simulink model "mVeh_fun_tbm"  (R2023b)
settings: Solver=FixedStepDiscrete  StartTime=0.0  StopTime=Parm_cnv_simulink_stopTime  FixedStep=Const_cnv_fundmt_stepSize  RelTol=1e-3  EnableMultiTasking=on
InitFcn:
  | preLoadFun
undefined symbols (not defined in the file or in its folder): Calib_pirelle_presSnr_x8, Calib_roadTriger_x6, Calib_tbm_brkBts_x8, Calib_tbm_ctr_x8, Calib_tbm_sensor_x4, Calib_tbm_strDistb_x8, Calib_tbm_supCtr_x8, CtrSet_tbm_enab_x8, IO397, Parm_tbmVeh_sig_max_numInvalid, Parm_tbmVeh_sig_tolerate_numInvalid
libraries: canmsglib x34, speedgoatlib_IO691 x19, MyLibrary x5, libtb_gen_canMsgCntr x5, speedgoatlib_fpga_analog_io x1, simulink x1, speedgoatlib_fpga x1, lib_decmp_CtrSet_tbm_enab_x8 x1, lib_decmp_Calib_tbm_brkPreTriger_x6 x1, lib_decmp_Calib_tbm_sensor_x4 x1
(part 2 of 3)

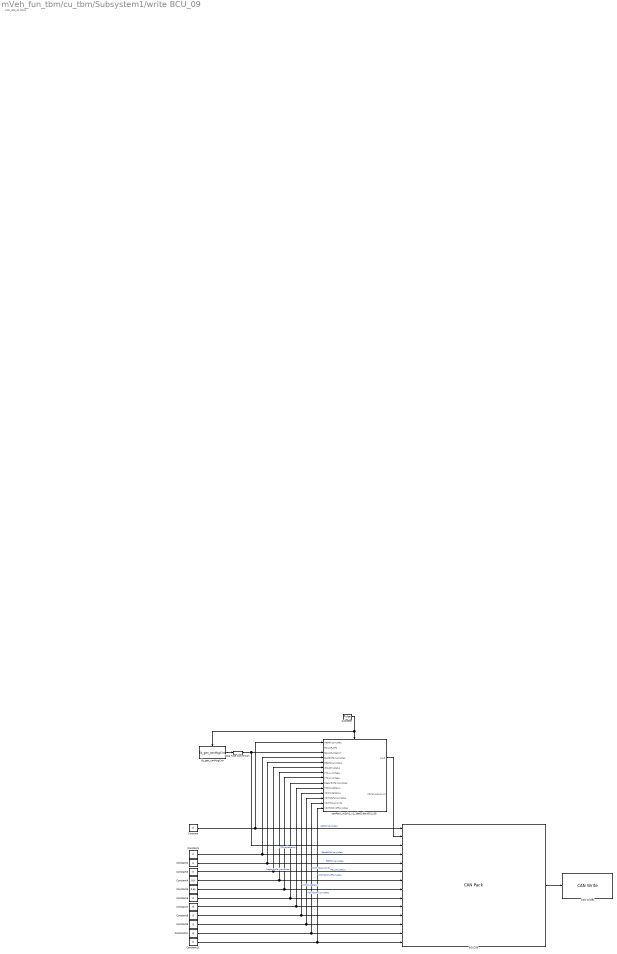
== system mVeh_fun_tbm/cu_tbm/Subsystem1/write BCU_09 ==
  note: ADC_EPS_01 20ms
  BCU_09 : canmsglib/CAN Pack  CANdbFile=C:\Users\bowen.zheng\Desktop\spdGoat_prj_20230315\spdGoat_prj_20230315\support\dbc\NIO_NT2_Chassis2_CAN_Official_Release_V_1_1_DA_02.dbc  MsgList=(none)  MsgName=BCU_09  MsgIDType=Standard (11-bit identifier)  MsgIdentifier=591  MsgLength=8  Remote=off  ApplyMinMax=off  BusOutput=off  SignalInfo={'ABSFailLampReq','37','1','BE','unsigned','Standard','0','1','0','0','1';'BCU_09_CRC','0','8','BE','unsigned','Standard','0','1','0','0','255';'BCU_09_MsgCntr','12','4','BE','unsigned','Standard','0','1','0','0','15';'BascBrkFailLampReq','32','2','BE','unsigned','Standard','0','1','0','0','3';'EBDFailLampReq','34','1','BE','unsigned','Standard','0','1','0','0','1';'IPB_CST_Status','38','2','BE','unsigned','Standard','0','1','0','0','3';'PTS_1_Voltage','17','9','BE','unsigned','Standard','0','0.01','-0.5','-0.5','4.61';'PTS_2_Voltage','24','9','BE','unsigned','Standard','0','0.01','-0.5','-0.5','4.61';'RegenBrkFailLampReq','10','1','BE','unsigned','Standard','0','1','0','0','1';'TCSModeStatus','45','3','BE','unsigned','Standard','0','1','0','0','7';'VDCModeStatus','42','3','BE','unsigned','Standard','0','1','0','0','7';'VDCTCSFailLampReq','36','1','BE','unsigned','Standard','0','1','0','0','1';'VDCTCSLampInfo','35','1','BE','unsigned','Standard','0','1','0','0','1';'VDCTCSOnOfflampReq','11','1','BE','unsigned','Standard','0','1','0','0','1'}
      settings: DataFormat=CANdb specified signals
  CAN Write1 : speedgoatlib_IO691/CAN Write  id=2  ts=0.1  channel=2  messageType=CAN  enableStatusPort=off  canType=CAN (HS)  initValues=[691 2 0.1 1 1 1 0]
  Constant{,1..3,6..11} (10 alike) : Constant  Value=0  OutDataTypeStr=single
  Constant4 : Constant  Value=0.9  OutDataTypeStr=single
  Constant5 : Constant  Value=0.44  OutDataTypeStr=single
  Data Type Conversion : DataTypeConversion  OutDataTypeStr=single  RndMeth=Nearest  SaturateOnIntegerOverflow=off
  canPack_nt2ch2_v1_1da02.dbc:BCU_09 : Subsystem
  lib_gen_canMsgCntr : libtb_gen_canMsgCntr/lib_gen_canMsgCntr  SystemSampleTime=-1  VariantActivationTime=update diagram  AllowFlexibleInterface=on  Latency=0  AutoFrameSizeCalculation=off
  pulseGen : DiscretePulseGenerator  PulseType=Time based  Period=0.1  PulseWidth=50
  wires:
  BCU_09/1 -> CAN Write1/1
  lib_gen_canMsgCntr/1 -> Data Type Conversion/1
  Constant/1 -> canPack_nt2ch2_v1_1da02.dbc:BCU_09/1(ABSFailLampReq), BCU_09/1  "ABSFailLampReq"
  Constant1/1 -> canPack_nt2ch2_v1_1da02.dbc:BCU_09/4(BascBrkFailLampReq), BCU_09/4  "BascBrkFailLampReq"
  Constant2/1 -> canPack_nt2ch2_v1_1da02.dbc:BCU_09/5(EBDFailLampReq), BCU_09/5  "EBDFailLampReq"
  Constant3/1 -> canPack_nt2ch2_v1_1da02.dbc:BCU_09/6(IPB_CST_Status), BCU_09/6  "IPB_CST_Status"
  Constant4/1 -> canPack_nt2ch2_v1_1da02.dbc:BCU_09/7(PTS_1_Voltage), BCU_09/7
  Constant5/1 -> canPack_nt2ch2_v1_1da02.dbc:BCU_09/8(PTS_2_Voltage), BCU_09/8
  Constant6/1 -> canPack_nt2ch2_v1_1da02.dbc:BCU_09/9(RegenBrkFailLampReq), BCU_09/9  "RegenBrkFailLampReq"
  Constant7/1 -> canPack_nt2ch2_v1_1da02.dbc:BCU_09/10(TCSModeStatus), BCU_09/10  "TCSModeStatus"
  Constant8/1 -> canPack_nt2ch2_v1_1da02.dbc:BCU_09/11(VDCModeStatus), BCU_09/11  "VDCModeStatus"
  Constant9/1 -> BCU_09/12, canPack_nt2ch2_v1_1da02.dbc:BCU_09/12(VDCTCSFailLampReq)  "VDCTCSFailLampReq"
  Constant10/1 -> canPack_nt2ch2_v1_1da02.dbc:BCU_09/13(VDCTCSLampInfo), BCU_09/13  "VDCTCSLampInfo"
  Constant11/1 -> canPack_nt2ch2_v1_1da02.dbc:BCU_09/14(VDCTCSOnOfflampReq), BCU_09/14  "VDCTCSOnOfflampReq"
  pulseGen/1 -> lib_gen_canMsgCntr/Trigger, canPack_nt2ch2_v1_1da02.dbc:BCU_09/Trigger
  Data Type Conversion/1 -> BCU_09/3, canPack_nt2ch2_v1_1da02.dbc:BCU_09/3(BCU_09_MsgCntr)
  canPack_nt2ch2_v1_1da02.dbc:BCU_09/1(crc_8) -> BCU_09/2

== system mVeh_fun_tbm/cu_tbm/Subsystem1/write VCU_14 ==
  note: ADC_EPS_01 20ms
  note: VCU_14 10ms
  cmd_brk_4whPres : Inport
  Bus Selector : BusSelector  OutputSignals=BTS_Active,BTS_BrakeTar_FL,BTS_BrakeTar_FR,BTS_BrakeTar_RL,BTS_BrakeTar_RR,VCU_14_CRC,VCU_14_MsgCntr
  CAN Write1 : speedgoatlib_IO691/CAN Write  id=2  ts=0.01  channel=2  messageType=CAN  enableStatusPort=off  canType=CAN (HS)  initValues=[691 2 0.01 1 1 1 0]
  Data Type Conversion : DataTypeConversion  OutDataTypeStr=single  RndMeth=Nearest  SaturateOnIntegerOverflow=off
  VCU_14*1 : canmsglib/CAN Pack  CANdbFile=.\support\dbc\NIO_NT2_Chassis2_CAN_Official_Release_V_1_1_DA_02.dbc  MsgList=VCU_14  MsgName=VCU_14  MsgIDType=Standard (11-bit identifier)  MsgIdentifier=75  MsgLength=8  Remote=off  ApplyMinMax=off  BusOutput=off  SignalInfo={'BTS_Active','23','1','BE','unsigned','Standard','0','1','0','0','1';'BTS_BrakeTar_FL','16','7','BE','unsigned','Standard','0','1','0','0','127';'BTS_BrakeTar_FR','25','7','BE','unsigned','Standard','0','1','0','0','127';'BTS_BrakeTar_RL','34','7','BE','unsigned','Standard','0','1','0','0','127';'BTS_BrakeTar_RR','43','7','BE','unsigned','Standard','0','1','0','0','127';'VCU_14_CRC','0','8','BE','unsigned','Standard','0','1','0','0','255';'VCU_14_MsgCntr','12','4','BE','unsigned','Standard','0','1','0','0','15'}
      settings: DataFormat=CANdb specified signals
  canPack_nt2ch2_v1_1da02.dbc:VCU_14 : Subsystem
  lib_gen_canMsgCntr : libtb_gen_canMsgCntr/lib_gen_canMsgCntr  SystemSampleTime=-1  VariantActivationTime=update diagram  AllowFlexibleInterface=on  Latency=0  AutoFrameSizeCalculation=off
  pulseGen : DiscretePulseGenerator  PulseType=Time based  Period=0.01  PulseWidth=50
  wires:
  canPack_nt2ch2_v1_1da02.dbc:VCU_14/1(crc_8) -> VCU_14*1/6
  VCU_14*1/1 -> CAN Write1/1
  cmd_brk_4whPres/1 -> Bus Selector/1
  pulseGen/1 -> canPack_nt2ch2_v1_1da02.dbc:VCU_14/Trigger, lib_gen_canMsgCntr/Trigger
  lib_gen_canMsgCntr/1 -> Data Type Conversion/1
  Bus Selector/1 -> canPack_nt2ch2_v1_1da02.dbc:VCU_14/1(BTS_Active), VCU_14*1/1  "<BTS_Active>"
  Bus Selector/6 -> ?  "<VCU_14_CRC>"
  Bus Selector/7 -> ?  "<VCU_14_MsgCntr>"
  Data Type Conversion/1 -> canPack_nt2ch2_v1_1da02.dbc:VCU_14/7(VCU_14_MsgCntr), VCU_14*1/7
  Bus Selector/2 -> canPack_nt2ch2_v1_1da02.dbc:VCU_14/2(BTS_BrakeTar_FL), VCU_14*1/2  "<BTS_BrakeTar_FL>"
  Bus Selector/3 -> canPack_nt2ch2_v1_1da02.dbc:VCU_14/3(BTS_BrakeTar_FR), VCU_14*1/3  "<BTS_BrakeTar_FR>"
  Bus Selector/4 -> canPack_nt2ch2_v1_1da02.dbc:VCU_14/4(BTS_BrakeTar_RL), VCU_14*1/4  "<BTS_BrakeTar_RL>"
  Bus Selector/5 -> canPack_nt2ch2_v1_1da02.dbc:VCU_14/5(BTS_BrakeTar_RR), VCU_14*1/5  "<BTS_BrakeTar_RR>"

== system mVeh_fun_tbm/cu_tbm/asm_canMsg/to_bcu_bts ==
  bts_enab : Inport
  cu_tbm : Inport  Port=2
  Bus Selector : BusSelector  OutputSignals=btsSimuDrBrk_actv,btsSimuDrBrk_mcp,tbmModfBrk_actv_4w,tbmModfBrk_pTgt_4w
  Data Type Conversion : DataTypeConversion  OutDataTypeStr=single  RndMeth=Nearest  SaturateOnIntegerOverflow=off
  Demux : Demux
  MATLAB Function : MATLAB Function  TreatAsAtomicUnit=on
  Rate Transition : RateTransition
  bus_VCU_14 : BusCreator  Inputs=7
  bus_to_ch2_VCU_14 : Outport
  wires:
  cu_tbm/1 -> Bus Selector/1
  ? -> bus_VCU_14/6  "VCU_14_CRC"
  ? -> bus_VCU_14/7  "VCU_14_MsgCntr"
  Demux/1 -> bus_VCU_14/2  "BTS_BrakeTar_FL"
  Demux/3 -> bus_VCU_14/4  "BTS_BrakeTar_RL"
  Data Type Conversion/1 -> bus_VCU_14/1  "BTS_Active"
  bus_VCU_14/1 -> bus_to_ch2_VCU_14/1  "bus_to_ch2_VCU_14"
  Demux/2 -> bus_VCU_14/3  "BTS_BrakeTar_FR"
  Demux/4 -> bus_VCU_14/5  "BTS_BrakeTar_RR"
  Bus Selector/1 -> MATLAB Function/2(btsSimuDrBrk_actv)  "<btsSimuDrBrk_actv>"
  MATLAB Function/1(btsCtr_actv) -> Rate Transition/1
  Bus Selector/3 -> MATLAB Function/4(tbmModfBrk_actv_4w)  "<tbmModfBrk_actv_4w>"
  Bus Selector/4 -> MATLAB Function/5(tbmModfBrk_pTgt_4w)  "<tbmModfBrk_pTgt_4w>"
  Bus Selector/2 -> MATLAB Function/3(btsSimuDrBrk_pTgt_4w)  "<btsSimuDrBrk_mcp>"
  MATLAB Function/2(bts_pTgt_4w) -> Demux/1  "bts_pTgt_4w"
  bts_enab/1 -> MATLAB Function/1(bts_enab)
  Rate Transition/1 -> Data Type Conversion/1

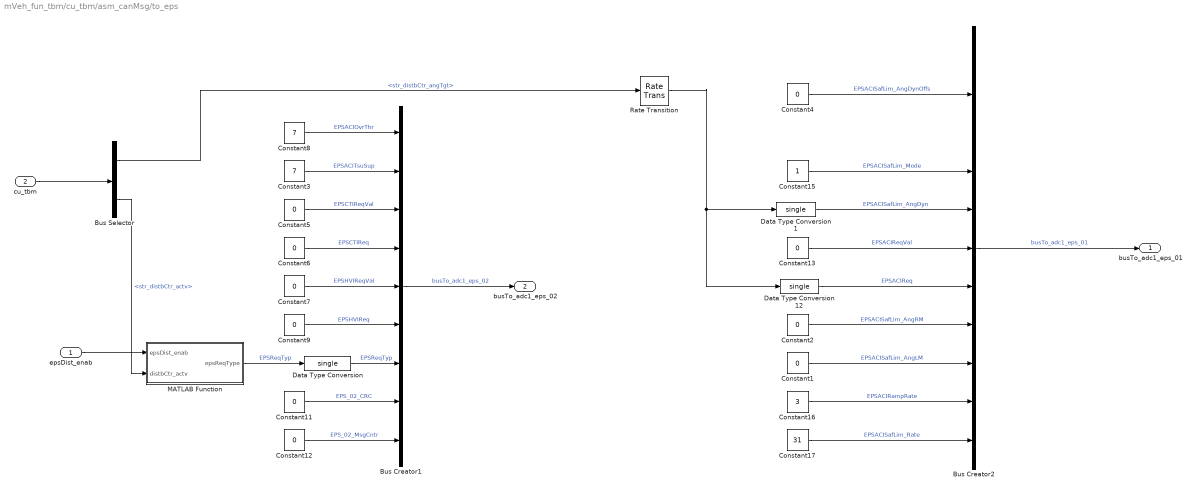
== system mVeh_fun_tbm/cu_tbm/asm_canMsg/to_eps ==
  epsDist_enab : Inport
  cu_tbm : Inport  Port=2
  Bus Creator1 : BusCreator  Inputs=9
  Bus Creator2 : BusCreator  Inputs=11
  Bus Selector : BusSelector  OutputSignals=str_distbCtr_angTgt,str_distbCtr_actv
  Constant{1..2,4..7,9,11..13} (10 alike) : Constant  Value=0  OutDataTypeStr=single
  Constant15 : Constant  OutDataTypeStr=single
  Constant16 : Constant  Value=3  OutDataTypeStr=single
  Constant17 : Constant  Value=31  OutDataTypeStr=single
  Constant3 : Constant  Value=7  OutDataTypeStr=single
  Constant8 : Constant  Value=7  OutDataTypeStr=single
  Data Type Conversion : DataTypeConversion  OutDataTypeStr=single  RndMeth=Nearest  SaturateOnIntegerOverflow=off
  Data Type Conversion1 : DataTypeConversion  OutDataTypeStr=single  RndMeth=Nearest  SaturateOnIntegerOverflow=off
  Data Type Conversion12 : DataTypeConversion  OutDataTypeStr=single  RndMeth=Nearest  SaturateOnIntegerOverflow=off
  MATLAB Function : MATLAB Function  TreatAsAtomicUnit=on
  Rate Transition : RateTransition
  busTo_adc1_eps_01 : Outport
  busTo_adc1_eps_02 : Outport  Port=2
  wires:
  ? -> Bus Creator2/3  "EPS_01_MsgCntr"
  Bus Selector/1 -> Rate Transition/1  "<str_distbCtr_angTgt>"
  Constant9/1 -> Bus Creator1/6  "EPSHVIReq"
  Constant11/1 -> Bus Creator1/8  "EPS_02_CRC"
  ? -> Bus Creator2/1  "EPS_01_CRC"
  Constant2/1 -> Bus Creator2/8  "EPSACISafLim_AngRM"
  MATLAB Function/1(epsReqType) -> Data Type Conversion/1  "EPSReqTyp"
  Constant17/1 -> Bus Creator2/11  "EPSACISafLim_Rate"
  Data Type Conversion1/1 -> Bus Creator2/5  "EPSACISafLim_AngDyn"
  Constant12/1 -> Bus Creator1/9  "EPS_02_MsgCntr"
  Constant1/1 -> Bus Creator2/9  "EPSACISafLim_AngLM"
  Bus Creator2/1 -> busTo_adc1_eps_01/1  "busTo_adc1_eps_01"
  Constant7/1 -> Bus Creator1/5  "EPSHVIReqVal"
  Constant6/1 -> Bus Creator1/4  "EPSCTIReq"
  Data Type Conversion12/1 -> Bus Creator2/7  "EPSACIReq"
  Constant13/1 -> Bus Creator2/6  "EPSACIReqVal"
  Constant16/1 -> Bus Creator2/10  "EPSACIRampRate"
  Constant3/1 -> Bus Creator1/2  "EPSACITsuSup"
  Constant8/1 -> Bus Creator1/1  "EPSACIOvrThr"
  Bus Creator1/1 -> busTo_adc1_eps_02/1  "busTo_adc1_eps_02"
  Constant5/1 -> Bus Creator1/3  "EPSCTIReqVal"
  Constant4/1 -> Bus Creator2/2  "EPSACISafLim_AngDynOffs"
  Constant15/1 -> Bus Creator2/4  "EPSACISafLim_Mode"
  cu_tbm/1 -> Bus Selector/1
  Bus Selector/2 -> MATLAB Function/2(distbCtr_actv)  "<str_distbCtr_actv>"
  epsDist_enab/1 -> MATLAB Function/1(epsDist_enab)
  Data Type Conversion/1 -> Bus Creator1/7  "EPSReqTyp"
  Rate Transition/1 -> Data Type Conversion12/1, Data Type Conversion1/1

== system mVeh_fun_tbm/cu_tbm/asm_canMsg/to_suspension ==
  suspCtr_enab : Inport
  cu_tbm : Inport  Port=2
  0: dump 2whls simutaniously : Constant  Value=0  OutDataTypeStr=single
  Bus Creator : BusCreator  Inputs=10
  Bus Selector : BusSelector  OutputSignals=susp_ctrActv_4w,susp_pTgt_4w
  Constant1 : Constant  Value=0  OutDataTypeStr=single
  Demux : Demux
  Demux1 : Demux
  MATLAB Function : MATLAB Function  TreatAsAtomicUnit=on
  RT{1..2,4..5} (4 alike) : RateTransition  OutPortSampleTime=0.001
  busTo_ch1_tbm_02 : Outport
  wires:
  cu_tbm/1 -> Bus Selector/1
  0: dump 2whls simutaniously/1 -> Bus Creator/5  "springID"
  Demux1/4 -> Bus Creator/4  "LeakActv_spring4"
  Demux/2 -> Bus Creator/7  "LeakTargPres_spring2"
  Demux/3 -> Bus Creator/8  "LeakTargPres_spring3"
  Demux/4 -> Bus Creator/9  "LeakTargPres_spring4"
  Demux1/1 -> Bus Creator/1  "LeakActv_spring1"
  Constant1/1 -> Bus Creator/10  "reserved"
  Demux1/2 -> Bus Creator/2  "LeakActv_spring2"
  Demux1/3 -> Bus Creator/3  "LeakActv_spring3"
  Demux/1 -> Bus Creator/6  "LeakTargPres_spring1"
  Bus Creator/1 -> busTo_ch1_tbm_02/1  "busTo_ch1_tbm_02"
  Bus Selector/2 -> RT5/1  "<susp_pTgt_4w>"
  Bus Selector/1 -> RT1/1  "<susp_ctrActv_4w>"
  MATLAB Function/1(suspCtr_actv_4w) -> RT4/1
  suspCtr_enab/1 -> RT2/1
  RT2/1 -> MATLAB Function/1(suspCtr_enab)
  RT1/1 -> MATLAB Function/2(suspCtr_actv_4w_in)
  RT5/1 -> Demux/1
  RT4/1 -> Demux1/1

== system mVeh_fun_tbm/cu_tbm/CAN Receive Unpack/Subsystem/ADC_Waypoint1 ==
  In1 : Inport
  ADC_Waypoint01 : canmsglib/CAN Unpack  CANdbFile=C:\Users\bowen.zheng\Desktop\spdGoat_prj_20230605\spdGoat_prj_20230605\support\dbc\NIO_NT2_Chassis2_CAN_Official_Release_V_1_1_DA_02.dbc  MsgList=ADC1_WayPoint01  MsgName=ADC1_WayPoint01  MsgIDType=Standard (11-bit identifier)  MsgIdentifier=214  MsgLength=8  SignalInfo={'LD_Confidence_1','24','4','BE','unsigned','Standard','0','0.1','0','0','1.5';'LD_First_End_1','51','7','BE','unsigned','Standard','0','1','0','0','127';'LD_First_Start_1','16','8','BE','unsigned','Standard','0','0.1','0','0','25.5';'LD_First_Type_1','28','4','BE','unsigned','Standard','0','1','0','0','15';'LD_Line_First_C0_1','56','11','BE','unsigned','Standard','0','0.01','-10.24','-10.24','10.23';'LD_Line_First_C1_1','43','13','BE','unsigned','Standard','0','0.0001','-0.4096','-0.4096','0.4095';'LD_Line_First_C2_1','0','8','BE','unsigned','Standard','0','0.0001','-0.0128','-0.0128','0.0127';'LD_Line_First_C3_1','8','8','BE','unsigned','Standard','0','1e-06','-0.000128','-0.000128','0.000127'}  IDPort=off  TimestampPort=off  ErrorPort=off  RemotePort=off  LengthPort=off  StatusPort=off  ApplyMinMax=off
      settings: DataFormat=CANdb specified signals
  LD_Confidence_1 : Outport
  LD_Line_First_C0_1 : Outport  Port=2
  wires:
  In1/1 -> ADC_Waypoint01/1
  ADC_Waypoint01/1 -> LD_Confidence_1/1  "LD_Confidence_1"
  ADC_Waypoint01/5 -> LD_Line_First_C0_1/1  "LD_Line_First_C0_1"

== system mVeh_fun_tbm/cu_tbm/CAN Receive Unpack/Subsystem/ADC_Waypoint2 ==
  In1 : Inport
  ADC_Waypoint01 : canmsglib/CAN Unpack  CANdbFile=C:\Users\bowen.zheng\Desktop\spdGoat_prj_20230605\spdGoat_prj_20230605\support\dbc\NIO_NT2_Chassis2_CAN_Official_Release_V_1_1_DA_02.dbc  MsgList=ADC1_WayPoint02  MsgName=ADC1_WayPoint02  MsgIDType=Standard (11-bit identifier)  MsgIdentifier=215  MsgLength=8  SignalInfo={'LD_Confidence_2','24','4','BE','unsigned','Standard','0','0.1','0','0','1.5';'LD_First_End_2','51','7','BE','unsigned','Standard','0','1','0','0','127';'LD_First_Start_2','16','8','BE','unsigned','Standard','0','0.1','0','0','25.5';'LD_First_Type_2','28','4','BE','unsigned','Standard','0','1','0','0','15';'LD_Line_First_C0_2','56','11','BE','unsigned','Standard','0','0.01','-10.24','-10.24','10.23';'LD_Line_First_C1_2','43','13','BE','unsigned','Standard','0','0.0001','-0.4096','-0.4096','0.4095';'LD_Line_First_C2_2','0','8','BE','unsigned','Standard','0','0.0001','-0.0128','-0.0128','0.0127';'LD_Line_First_C3_2','8','8','BE','unsigned','Standard','0','1e-06','-0.000128','-0.000128','0.000127'}  IDPort=off  TimestampPort=off  ErrorPort=off  RemotePort=off  LengthPort=off  StatusPort=off  ApplyMinMax=off
      settings: DataFormat=CANdb specified signals
  LD_Confidence_2 : Outport
  LD_Line_First_C0_2 : Outport  Port=2
  wires:
  In1/1 -> ADC_Waypoint01/1
  ADC_Waypoint01/1 -> LD_Confidence_2/1  "LD_Confidence_2"
  ADC_Waypoint01/5 -> LD_Line_First_C0_2/1  "LD_Line_First_C0_2"

== system mVeh_fun_tbm/cu_tbm/CAN Receive Unpack/Subsystem/ADC_Waypoint3 ==
  In1 : Inport
  ADC_Waypoint01 : canmsglib/CAN Unpack  CANdbFile=C:\Users\bowen.zheng\Desktop\spdGoat_prj_20230605\spdGoat_prj_20230605\support\dbc\NIO_NT2_Chassis2_CAN_Official_Release_V_1_1_DA_02.dbc  MsgList=ADC1_WayPoint03  MsgName=ADC1_WayPoint03  MsgIDType=Standard (11-bit identifier)  MsgIdentifier=216  MsgLength=8  SignalInfo={'LD_Confidence_3','24','4','BE','unsigned','Standard','0','0.1','0','0','1.5';'LD_First_End_3','51','7','BE','unsigned','Standard','0','1','0','0','127';'LD_First_Start_3','16','8','BE','unsigned','Standard','0','0.1','0','0','25.5';'LD_First_Type_3','28','4','BE','unsigned','Standard','0','1','0','0','15';'LD_Line_First_C0_3','56','11','BE','unsigned','Standard','0','0.01','-10.24','-10.24','10.23';'LD_Line_First_C1_3','43','13','BE','unsigned','Standard','0','0.0001','-0.4096','-0.4096','0.4095';'LD_Line_First_C2_3','0','8','BE','unsigned','Standard','0','0.0001','-0.0128','-0.0128','0.0127';'LD_Line_First_C3_3','8','8','BE','unsigned','Standard','0','1e-06','-0.000128','-0.000128','0.000127'}  IDPort=off  TimestampPort=off  ErrorPort=off  RemotePort=off  LengthPort=off  StatusPort=off  ApplyMinMax=off
      settings: DataFormat=CANdb specified signals
  LD_Confidence_3 : Outport
  LD_Line_First_C0_3 : Outport  Port=2
  wires:
  In1/1 -> ADC_Waypoint01/1
  ADC_Waypoint01/1 -> LD_Confidence_3/1  "LD_Confidence_3"
  ADC_Waypoint01/5 -> LD_Line_First_C0_3/1  "LD_Line_First_C0_3"

== system mVeh_fun_tbm/cu_tbm/CAN Receive Unpack/Subsystem/ADC_Waypoint4 ==
  In1 : Inport
  ADC_Waypoint01 : canmsglib/CAN Unpack  CANdbFile=C:\Users\bowen.zheng\Desktop\spdGoat_prj_20230605\spdGoat_prj_20230605\support\dbc\NIO_NT2_Chassis2_CAN_Official_Release_V_1_1_DA_02.dbc  MsgList=ADC1_WayPoint04  MsgName=ADC1_WayPoint04  MsgIDType=Standard (11-bit identifier)  MsgIdentifier=217  MsgLength=8  SignalInfo={'LD_Confidence_4','24','4','BE','unsigned','Standard','0','0.1','0','0','1.5';'LD_First_End_4','51','7','BE','unsigned','Standard','0','1','0','0','127';'LD_First_Start_4','16','8','BE','unsigned','Standard','0','0.1','0','0','25.5';'LD_First_Type_4','28','4','BE','unsigned','Standard','0','1','0','0','15';'LD_Line_First_C0_4','56','11','BE','unsigned','Standard','0','0.01','-10.24','-10.24','10.23';'LD_Line_First_C1_4','43','13','BE','unsigned','Standard','0','0.0001','-0.4096','-0.4096','0.4095';'LD_Line_First_C2_4','0','8','BE','unsigned','Standard','0','0.0001','-0.0128','-0.0128','0.0127';'LD_Line_First_C3_4','8','8','BE','unsigned','Standard','0','1e-06','-0.000128','-0.000128','0.000127'}  IDPort=off  TimestampPort=off  ErrorPort=off  RemotePort=off  LengthPort=off  StatusPort=off  ApplyMinMax=off
      settings: DataFormat=CANdb specified signals
  LD_Confidence_4 : Outport
  LD_Line_First_C0_4 : Outport  Port=2
  wires:
  In1/1 -> ADC_Waypoint01/1
  ADC_Waypoint01/1 -> LD_Confidence_4/1  "LD_Confidence_4"
  ADC_Waypoint01/5 -> LD_Line_First_C0_4/1  "LD_Line_First_C0_4"

== system mVeh_fun_tbm/cu_tbm/Chassis 1 read/Subsystem/ACM_02 ==
  In1 : Inport
  Chassis 1 ACM_02 : canmsglib/CAN Unpack  CANdbFile=.\support\dbc\NIO_NT2_Chassis1_CAN_Official_Release_V_1_1_DA_02.dbc  MsgList=ACM_02  MsgName=ACM_02  MsgIDType=Standard (11-bit identifier)  MsgIdentifier=61  MsgLength=6  SignalInfo={'ACM_02_CRC','0','8','BE','unsigned','Standard','0','1','0','0','255';'ACM_02_MsgCntr','12','4','BE','unsigned','Standard','0','1','0','0','15';'LatA','40','16','BE','unsigned','Standard','0','0.001','-2','-2','2';'LatAValSts','8','2','BE','unsigned','Standard','0','1','0','0','3';'YawRate','24','16','BE','unsigned','Standard','0','0.01','-180','-180','180';'YawRateValSts','10','2','BE','unsigned','Standard','0','1','0','0','3'}  IDPort=off  TimestampPort=off  ErrorPort=off  RemotePort=off  LengthPort=off  StatusPort=off  ApplyMinMax=off
      settings: DataFormat=CANdb specified signals
  Terminator : Terminator
  Terminator1 : Terminator
  wires:
  In1/1 -> Chassis 1 ACM_02/1
  Chassis 1 ACM_02/3 -> Terminator/1  "ACM_02_LatA"
  Chassis 1 ACM_02/5 -> Terminator1/1  "ACM_02_YawRate"

== system mVeh_fun_tbm/cu_tbm/Chassis 1 read/Subsystem/ACM_03 ==
  In1 : Inport
  Chassis 1 ACM_03 : canmsglib/CAN Unpack  CANdbFile=.\support\dbc\NIO_NT2_Chassis1_CAN_Official_Release_V_1_1_DA_02.dbc  MsgList=ACM_03  MsgName=ACM_03  MsgIDType=Standard (11-bit identifier)  MsgIdentifier=62  MsgLength=4  SignalInfo={'ACM_03_CRC','0','8','BE','unsigned','Standard','0','1','0','0','255';'ACM_03_MsgCntr','12','4','BE','unsigned','Standard','0','1','0','0','15';'AxAyYrsCalSts','8','2','BE','unsigned','Standard','0','1','0','0','3';'LgtA','24','16','BE','unsigned','Standard','0','0.001','-2','-2','2';'LgtAValSts','10','2','BE','unsigned','Standard','0','1','0','0','3'}  IDPort=off  TimestampPort=off  ErrorPort=off  RemotePort=off  LengthPort=off  StatusPort=off  ApplyMinMax=off
      settings: DataFormat=CANdb specified signals
  Terminator1 : Terminator
  wires:
  In1/1 -> Chassis 1 ACM_03/1
  Chassis 1 ACM_03/4 -> Terminator1/1  "ACM_03_LgtA"

== system mVeh_fun_tbm/cu_tbm/Chassis 1 read/Subsystem/BCU_01 ==
  In1 : Inport
  Chassis 1 BCU_01 : canmsglib/CAN Unpack  CANdbFile=.\support\dbc\NIO_NT2_Chassis1_CAN_Official_Release_V_1_1_DA_02.dbc  MsgList=BCU_01  MsgName=BCU_01  MsgIDType=Standard (11-bit identifier)  MsgIdentifier=88  MsgLength=6  SignalInfo={'BCU_01_CRC','0','8','BE','unsigned','Standard','0','1','0','0','255';'BCU_01_MsgCntr','12','4','BE','unsigned','Standard','0','1','0','0','15';'WhlSpdFrntLe','24','13','BE','unsigned','Standard','0','0.05625','0','0','360';'WhlSpdFrntLeMovgDir','37','2','BE','unsigned','Standard','0','1','0','0','3';'WhlSpdFrntLeSts','10','2','BE','unsigned','Standard','0','1','0','0','3';'WhlSpdFrntRi','40','13','BE','unsigned','Standard','0','0.05625','0','0','360';'WhlSpdFrntRiMovgDir','21','2','BE','unsigned','Standard','0','1','0','0','3';'WhlSpdFrntRiSts','8','2','BE','unsigned','Standard','0','1','0','0','3'}  IDPort=off  TimestampPort=off  ErrorPort=off  RemotePort=off  LengthPort=off  StatusPort=off  ApplyMinMax=off
      settings: DataFormat=CANdb specified signals
  Terminator1 : Terminator
  Terminator2 : Terminator
  wires:
  In1/1 -> Chassis 1 BCU_01/1
  Chassis 1 BCU_01/3 -> Terminator2/1  "BCU_01_WhlSpdFrntLe"
  Chassis 1 BCU_01/6 -> Terminator1/1  "BCU_01_WhlSpdFrntRi"

== system mVeh_fun_tbm/cu_tbm/Chassis 1 read/Subsystem/BCU_02 ==
  In1 : Inport
  Chassis 1 BCU_02 : canmsglib/CAN Unpack  CANdbFile=.\support\dbc\NIO_NT2_Chassis1_CAN_Official_Release_V_1_1_DA_02.dbc  MsgList=BCU_02  MsgName=BCU_02  MsgIDType=Standard (11-bit identifier)  MsgIdentifier=89  MsgLength=6  SignalInfo={'BCU_02_CRC','0','8','BE','unsigned','Standard','0','1','0','0','255';'BCU_02_MsgCntr','12','4','BE','unsigned','Standard','0','1','0','0','15';'WhlSpdReLe','24','13','BE','unsigned','Standard','0','0.05625','0','0','360';'WhlSpdReLeMovgDir','21','2','BE','unsigned','Standard','0','1','0','0','3';'WhlSpdReLeSts','10','2','BE','unsigned','Standard','0','1','0','0','3';'WhlSpdReRi','40','13','BE','unsigned','Standard','0','0.05625','0','0','360';'WhlSpdReRiMovgDir','37','2','BE','unsigned','Standard','0','1','0','0','3';'WhlSpdReRiSts','8','2','BE','unsigned','Standard','0','1','0','0','3'}  IDPort=off  TimestampPort=off  ErrorPort=off  RemotePort=off  LengthPort=off  StatusPort=off  ApplyMinMax=off
      settings: DataFormat=CANdb specified signals
  Terminator1 : Terminator
  Terminator2 : Terminator
  wires:
  In1/1 -> Chassis 1 BCU_02/1
  Chassis 1 BCU_02/3 -> Terminator2/1  "BCU_02_WhlSpdReLe"
  Chassis 1 BCU_02/6 -> Terminator1/1  "BCU_02_WhlSpdReRi"

== system mVeh_fun_tbm/cu_tbm/Chassis 1 read/Subsystem/BCU_04 ==
  In1 : Inport
  Bus Creator : BusCreator  Inputs=2
  Bus Creator1 : BusCreator  Inputs=2
  Chassis 1 BCU_04 : canmsglib/CAN Unpack  CANdbFile=.\support\dbc\NIO_NT2_Chassis1_CAN_Official_Release_V_1_1_DA_02.dbc  MsgList=BCU_04  MsgName=BCU_04  MsgIDType=Standard (11-bit identifier)  MsgIdentifier=91  MsgLength=8  SignalInfo={'BCUBrkLiReq','9','2','BE','unsigned','Standard','0','1','0','0','3';'BCU_04_CRC','0','8','BE','unsigned','Standard','0','1','0','0','255';'BCU_04_MsgCntr','12','4','BE','unsigned','Standard','0','1','0','0','15';'BCU_NoBrkF','8','1','BE','unsigned','Standard','0','1','0','0','1';'BCU_SupInfo','48','2','BE','unsigned','Standard','0','1','0','0','3';'BrkOverHeat','50','1','BE','unsigned','Standard','0','1','0','0','1';'BrkPedlSts','54','2','BE','unsigned','Standard','0','1','0','0','3';'BrkPedlTrvl','56','8','BE','unsigned','Standard','0','0.4','0','0','102';'BrkPedlTrvlCalSts','52','2','BE','unsigned','Standard','0','1','0','0','3';'BrkPress','47','9','BE','unsigned','Standard','0','1','-42.5','-42.5','425.5';'BrkPressOffset','42','5','BE','unsigned','Standard','0','1','-15','-15','15';'BrkPressOffsetValid','41','1','BE','unsigned','Standard','0','1','0','0','1';'BrkPressValid','40','1','BE','unsigned','Standard','0','1','0','0','1';'HAZReq','11','1','BE','unsigned','Standard','0','1','0','0','1';'IPB_TwoFoot_DriveWarning','51','1','BE','unsigned','Standard','0','1','0','0','1';'VehMovgDir','21','2','BE','unsigned','Standard','0','1','0','0','3';'VehSpd','24','13','BE','unsigned','Standard','0','0.05625','0','0','360';'VehSpdSts','23','1','BE','unsigned','Standard','0','1','0','0','1'}  IDPort=off  TimestampPort=off  ErrorPort=off  RemotePort=off  LengthPort=off  StatusPort=off  ApplyMinMax=off
      settings: DataFormat=CANdb specified signals
  Terminator{,1..4} (5 alike) : Terminator
  BCU_04_VehSpd_w_Validity : Outport
  BCU_04_BrkPedl_w_Sts : Outport  Port=2
  wires:
  Chassis 1 BCU_04/8 -> Terminator2/1  "BCU_04_BrkPedlTrvl"
  Chassis 1 BCU_04/3 -> Terminator/1  "BCU_04_MsgCntr"
  Chassis 1 BCU_04/2 -> Terminator1/1  "BCU_04_CRC"
  Chassis 1 BCU_04/7 -> Bus Creator1/1  "BCU_04_BrkPedlSts"
  Chassis 1 BCU_04/13 -> Terminator4/1  "BCU_04_BrkPressValid"
  Chassis 1 BCU_04/10 -> Terminator3/1  "BCU_04_BrkPress"
  Chassis 1 BCU_04/17 -> Bus Creator/1  "BCU_04_VehSpd"
  Chassis 1 BCU_04/18 -> Bus Creator/2  "BCU_04_VehSpdSts"
  Chassis 1 BCU_04/9 -> Bus Creator1/2  "BCU_04_BrkPedlTrvlCalSts"
  In1/1 -> Chassis 1 BCU_04/1
  Bus Creator/1 -> BCU_04_VehSpd_w_Validity/1
  Bus Creator1/1 -> BCU_04_BrkPedl_w_Sts/1

== system mVeh_fun_tbm/cu_tbm/Chassis 1 read/Subsystem/BCU_19 ==
  In1 : Inport
  Chassis 1 BCU_19 : canmsglib/CAN Unpack  CANdbFile=.\support\dbc\NIO_NT2_Chassis1_CAN_Official_Release_V_1_1_DA_02.dbc  MsgList=BCU_19  MsgName=BCU_19  MsgIDType=Standard (11-bit identifier)  MsgIdentifier=107  MsgLength=8  SignalInfo={'PSP_Pressure','56','12','BE','unsigned','Standard','0','0.05','-5','-5','199.75';'WheelBrkPFrntLe','12','12','BE','unsigned','Standard','0','0.1','0','0','409.5';'WheelBrkPFrntRi','16','12','BE','unsigned','Standard','0','0.1','0','0','409.5';'WheelBrkPReLe','36','12','BE','unsigned','Standard','0','0.1','0','0','409.5';'WheelBrkPReRi','40','12','BE','unsigned','Standard','0','0.1','0','0','409.5';'WheelBrkPReliabilityFrntLe','55','1','BE','unsigned','Standard','0','1','0','0','1';'WheelBrkPReliabilityFrntRi','54','1','BE','unsigned','Standard','0','1','0','0','1';'WheelBrkPReliabilityReLe','53','1','BE','unsigned','Standard','0','1','0','0','1';'WheelBrkPReliabilityReRi','52','1','BE','unsigned','Standard','0','1','0','0','1'}  IDPort=off  TimestampPort=off  ErrorPort=off  RemotePort=off  LengthPort=off  StatusPort=off  ApplyMinMax=off
      settings: DataFormat=CANdb specified signals
  Terminator{,1..3} (4 alike) : Terminator
  wires:
  In1/1 -> Chassis 1 BCU_19/1
  Chassis 1 BCU_19/2 -> Terminator/1  "BCU_19_WheelBrkPFrntLe"
  Chassis 1 BCU_19/3 -> Terminator1/1  "BCU_19_WheelBrkPFrntRi"
  Chassis 1 BCU_19/4 -> Terminator2/1  "BCU_19_WheelBrkPReLe"
  Chassis 1 BCU_19/5 -> Terminator3/1  "BCU_19_WheelBrkPReRi"

== system mVeh_fun_tbm/cu_tbm/Chassis 1 read/Subsystem/BGW_02 ==
  In1 : Inport
  Chassis 1 BGW_02 : canmsglib/CAN Unpack  CANdbFile=.\support\dbc\NIO_NT2_Chassis1_CAN_Official_Release_V_1_1_DA_02.dbc  MsgList=BGW_02  MsgName=BGW_02  MsgIDType=Standard (11-bit identifier)  MsgIdentifier=707  MsgLength=2  SignalInfo={'ComfEna','2','2','BE','unsigned','Standard','0','1','0','0','3';'FOTAHvPwrMgnt','0','2','BE','unsigned','Standard','0','1','0','0','3';'ImobEnaReq','14','2','BE','unsigned','Standard','0','1','0','0','3';'ImobSts','8','2','BE','unsigned','Standard','0','1','0','0','3';'KeyAuthSts','10','2','BE','unsigned','Standard','0','1','0','0','3';'KeyPrsntSts','12','2','BE','unsigned','Standard','0','1','0','0','3';'VehState','4','4','BE','unsigned','Standard','0','1','0','0','15'}  IDPort=off  TimestampPort=off  ErrorPort=off  RemotePort=off  LengthPort=off  StatusPort=off  ApplyMinMax=off
      settings: DataFormat=CANdb specified signals
  BGW_02_VehState : Outport
  wires:
  In1/1 -> Chassis 1 BGW_02/1
  Chassis 1 BGW_02/7 -> BGW_02_VehState/1  "BGW_02_VehState"

== system mVeh_fun_tbm/cu_tbm/Chassis 1 read/Subsystem/EPS_01 ==
  In1 : Inport
  Chassis 1 EPS_01 : canmsglib/CAN Unpack  CANdbFile=.\support\dbc\NIO_NT2_Chassis1_CAN_Official_Release_V_1_1_DA_02.dbc  MsgList=EPS1_01  MsgName=EPS1_01  MsgIDType=Standard (11-bit identifier)  MsgIdentifier=116  MsgLength=8  SignalInfo={'EPS1_01_CRC','0','8','BE','unsigned','Standard','0','1','0','0','255';'EPS1_01_MsgCntr','12','4','BE','unsigned','Standard','0','1','0','0','15';'EPS1_ADCACIOlAvl','55','1','BE','unsigned','Standard','0','1','0','0','1';'EPS1_ADCACIOrAvl','41','1','BE','unsigned','Standard','0','1','0','0','1';'EPS1_ADCCTIAvl','44','1','BE','unsigned','Standard','0','1','0','0','1';'EPS1_ADCHVIAvl','46','1','BE','unsigned','Standard','0','1','0','0','1';'EPS1_ActvExtIf','48','5','BE','unsigned','Standard','0','1','0','0','31';'EPS1_BCUCTIAvl','42','1','BE','unsigned','Standard','0','1','0','0','1';'EPS1_DrivingMod','10','2','BE','unsigned','Standard','0','1','0','0','3';'EPS1_OverRideSts','47','1','BE','unsigned','Standard','0','1','0','0','1';'EPS1_PinAng','32','15','BE','unsigned','Standard','0','0.1','-1638.4','-1638.4','1638.2';'EPS1_PinAngOffset','16','10','BE','unsigned','Standard','0','0.1','-51.2','-51.2','51.1';'EPS1_PinAngVal','31','1','BE','unsigned','Standard','0','1','0','0','1';'EPS1_RampSts','60','1','BE','unsigned','Standard','0','1','0','0','1';'EPS1_Sts','61','3','BE','unsigned','Standard','0','1','0','0','7';'EPS1_VMCACIOlAvl','54','1','BE','unsigned','Standard','0','1','0','0','1';'EPS1_VMCACIOrAvl','40','1','BE','unsigned','Standard','0','1','0','0','1';'EPS1_VMCCTIAvl','43','1','BE','unsigned','Standard','0','1','0','0','1';'EPS1_VMCHVIAvl','45','1','BE','unsigned','Standard','0','1','0','0','1';'EPS1_VMCMTIAvl','53','1','BE','unsigned','Standard','0','1','0','0','1';'EPS1_WarnLampReq','58','2','BE','unsigned','Standard','0','1','0','0','3'}  IDPort=off  TimestampPort=off  ErrorPort=off  RemotePort=off  LengthPort=off  StatusPort=off  ApplyMinMax=off
      settings: DataFormat=CANdb specified signals
  Terminator : Terminator
  Terminator1 : Terminator
  Terminator2 : Terminator
  wires:
  In1/1 -> Chassis 1 EPS_01/1
  Chassis 1 EPS_01/15 -> Terminator2/1  "EPS1_Sts"
  Chassis 1 EPS_01/11 -> Terminator1/1  "EPS1_PinAng"
  Chassis 1 EPS_01/7 -> Terminator/1  "EPS1_ActvExtIf"

== system mVeh_fun_tbm/cu_tbm/Chassis 1 read/Subsystem/EPS_02 ==
  In1 : Inport
  Chassis 1 EPS_02 : canmsglib/CAN Unpack  CANdbFile=.\support\dbc\NIO_NT2_Chassis1_CAN_Official_Release_V_1_1_DA_02.dbc  MsgList=EPS1_02  MsgName=EPS1_02  MsgIDType=Standard (11-bit identifier)  MsgIdentifier=117  MsgLength=8  SignalInfo={'EPS1_02_CRC','0','8','BE','unsigned','Standard','0','1','0','0','255';'EPS1_02_MsgCntr','12','4','BE','unsigned','Standard','0','1','0','0','15';'EPS1_ACIMotorTq','58','10','BE','unsigned','Standard','0','0.02','-10.24','-10.24','10.22';'EPS1_ACIMotorTqVal','52','1','BE','unsigned','Standard','0','1','0','0','1';'EPS1_EstRackForce','32','10','BE','unsigned','Standard','0','0.04','-20.48','-20.48','20.44';'EPS1_EstRackForceVal','28','1','BE','unsigned','Standard','0','1','0','0','1';'EPS1_SupInfo','26','2','BE','unsigned','Standard','0','1','0','0','3';'EPS1_Temperature','8','4','BE','unsigned','Standard','0','1','0','0','15';'EPS1_TorsBarTq','30','10','BE','unsigned','Standard','0','0.02','-10.24','-10.24','10.22';'EPS1_TorsBarTqVal','29','1','BE','unsigned','Standard','0','1','0','0','1';'EPS1_TotMotorTq','54','10','BE','unsigned','Standard','0','0.02','-10.24','-10.24','10.22';'EPS1_TotMotorTqVal','53','1','BE','unsigned','Standard','0','1','0','0','1'}  IDPort=off  TimestampPort=off  ErrorPort=off  RemotePort=off  LengthPort=off  StatusPort=off  ApplyMinMax=off
      settings: DataFormat=CANdb specified signals
  Terminator2 : Terminator
  wires:
  In1/1 -> Chassis 1 EPS_02/1
  Chassis 1 EPS_02/9 -> Terminator2/1  "EPS1_TorsBarTq"

== system mVeh_fun_tbm/cu_tbm/Chassis 1 read/Subsystem/PEUF_VCU_84 ==
  In1 : Inport
  Chassis 1 PEUF_VCU_84 : canmsglib/CAN Unpack  CANdbFile=C:\Users\bowen.zheng\Desktop\spdGoat_prj_20230322\spdGoat_prj_20230322\support\dbc\NIO_NT2_Chassis1_CAN_Official_Release_V_1_1_DA_02.dbc  MsgList=(none)  MsgName=PEUF_VCU_84  MsgIDType=Standard (11-bit identifier)  MsgIdentifier=132  MsgLength=8  SignalInfo={'PEUFDampSts','33','2','BE','unsigned','Standard','0','1','0','0','3';'PEUFFailrSts','37','3','BE','unsigned','Standard','0','1','0','0','7';'PEUFHeatCap','52','4','BE','unsigned','Standard','0','1','0','0','15';'PEUFMotActTq','8','15','BE','signed','Standard','0','0.125','0','-2048','2047.875';'PEUFMotActTqValid','7','1','BE','unsigned','Standard','0','1','0','0','1';'PEUFMotHoldSts','35','2','BE','unsigned','Standard','0','1','0','0','3';'PEUFMotSpd','24','16','BE','signed','Standard','0','1','0','-32768','32767';'PEUFMotSpdValid','32','1','BE','unsigned','Standard','0','1','0','0','1';'PEUF_SpdLimForFlt','40','8','BE','unsigned','Standard','0','1','0','0','255';'PEUF_VCU_84_CRC','56','8','BE','unsigned','Standard','0','1','0','0','255';'PEUF_VCU_84_MsgCntr','48','4','BE','unsigned','Standard','0','1','0','0','15'}  IDPort=off  TimestampPort=off  ErrorPort=off  RemotePort=off  LengthPort=off  StatusPort=off  ApplyMinMax=off
      settings: DataFormat=CANdb specified signals
  Terminator1 : Terminator
  wires:
  In1/1 -> Chassis 1 PEUF_VCU_84/1
  Chassis 1 PEUF_VCU_84/4 -> Terminator1/1  "PEUF_VCU_84_PEUFMotActTq"

== system mVeh_fun_tbm/cu_tbm/Chassis 1 read/Subsystem/PEUR_VCU_8C ==
  In1 : Inport
  Chassis 1 PEUR_VCU_8C : canmsglib/CAN Unpack  CANdbFile=C:\Users\bowen.zheng\Desktop\spdGoat_prj_20230322\spdGoat_prj_20230322\support\dbc\NIO_NT2_Chassis1_CAN_Official_Release_V_1_1_DA_02.dbc  MsgList=(none)  MsgName=PEUR_VCU_8C  MsgIDType=Standard (11-bit identifier)  MsgIdentifier=140  MsgLength=8  SignalInfo={'PEURDampSts','33','2','BE','unsigned','Standard','0','1','0','0','3';'PEURFailrSts','37','3','BE','unsigned','Standard','0','1','0','0','7';'PEURHeatCap','52','4','BE','unsigned','Standard','0','1','0','0','15';'PEURMotActTq','8','15','BE','signed','Standard','0','0.125','0','-2048','2047.875';'PEURMotActTqValid','7','1','BE','unsigned','Standard','0','1','0','0','1';'PEURMotHoldSts','35','2','BE','unsigned','Standard','0','1','0','0','3';'PEURMotSpd','24','16','BE','signed','Standard','0','1','0','-32768','32767';'PEURMotSpdValid','32','1','BE','unsigned','Standard','0','1','0','0','1';'PEUR_SpdLimForFlt','40','8','BE','unsigned','Standard','0','1','0','0','255';'PEUR_VCU_8C_CRC','56','8','BE','unsigned','Standard','0','1','0','0','255';'PEUR_VCU_8C_MsgCntr','48','4','BE','unsigned','Standard','0','1','0','0','15'}  IDPort=off  TimestampPort=off  ErrorPort=off  RemotePort=off  LengthPort=off  StatusPort=off  ApplyMinMax=off
      settings: DataFormat=CANdb specified signals
  Terminator1 : Terminator
  wires:
  In1/1 -> Chassis 1 PEUR_VCU_8C/1
  Chassis 1 PEUR_VCU_8C/4 -> Terminator1/1  "PEUR_VCU_8C_PEURMotActTq"

== system mVeh_fun_tbm/cu_tbm/Chassis 1 read/Subsystem/SCM_01 ==
  In1 : Inport
  Chassis 1 SCM_01 : canmsglib/CAN Unpack  CANdbFile=.\support\dbc\NIO_NT2_Chassis1_CAN_Official_Release_V_1_1_DA_02.dbc  MsgList=SCM_01  MsgName=SCM_01  MsgIDType=Standard (11-bit identifier)  MsgIdentifier=212  MsgLength=6  SignalInfo={'SCM_01_CRC','0','8','BE','unsigned','Standard','0','1','0','0','255';'SCM_01_MsgCntr','12','4','BE','unsigned','Standard','0','1','0','0','15';'SteerAgSnsrCalSts','11','1','BE','unsigned','Standard','0','1','0','0','1';'SteerAgSnsrFailSts','8','2','BE','unsigned','Standard','0','1','0','0','3';'SteerWhlAg','24','13','BE','unsigned','Standard','0','0.1','0','0','800';'SteerWhlAgAndSpdValid','10','1','BE','unsigned','Standard','0','1','0','0','1';'SteerWhlAgDir','21','1','BE','unsigned','Standard','0','1','0','0','1';'SteerWhlAgSpd','40','9','BE','unsigned','Standard','0','5','0','0','2550';'SteerWhlAgSpdDir','33','1','BE','unsigned','Standard','0','1','0','0','1'}  IDPort=off  TimestampPort=off  ErrorPort=off  RemotePort=off  LengthPort=off  StatusPort=off  ApplyMinMax=off
      settings: DataFormat=CANdb specified signals
  Terminator : Terminator
  Terminator1 : Terminator
  Terminator2 : Terminator
  wires:
  In1/1 -> Chassis 1 SCM_01/1
  Chassis 1 SCM_01/7 -> Terminator1/1  "SCM_01_SteerWhlAgDir"
  Chassis 1 SCM_01/5 -> Terminator/1  "SCM_01_SteerWhlAg"
  Chassis 1 SCM_01/8 -> Terminator2/1  "SCM_01_SteerWhlAgSpd"

== system mVeh_fun_tbm/cu_tbm/Chassis 1 read/Subsystem/VCU_02 ==
  In1 : Inport
  Chassis 1 VCU_02 : canmsglib/CAN Unpack  CANdbFile=C:\Users\bowen.zheng\Desktop\spdGoat_prj_20230322\spdGoat_prj_20230322\support\dbc\NIO_NT2_Chassis1_CAN_Official_Release_V_1_1_DA_02.dbc  MsgList=(none)  MsgName=VCU_02  MsgIDType=Standard (11-bit identifier)  MsgIdentifier=69  MsgLength=8  SignalInfo={'AccrPedlActPosn','40','8','BE','unsigned','Standard','0','0.392','0','0','99.96';'AccrPedlActPosnValid','54','1','BE','unsigned','Standard','0','1','0','0','1';'AccrPedlEfcPosn','32','8','BE','unsigned','Standard','0','0.392','0','0','99.96';'AccrPedlEfcPosnValid','55','1','BE','unsigned','Standard','0','1','0','0','1';'VCUAccrPedlOvrd','53','1','BE','unsigned','Standard','0','1','0','0','1';'VCUIntdFrntMotTq','8','15','BE','signed','Standard','0','0.125','0','-2048','2047.875';'VCUIntdFrntMotTqValid','7','1','BE','unsigned','Standard','0','1','0','0','1';'VCUIntdReMotTq','24','15','BE','signed','Standard','0','0.125','0','-2048','2047.875';'VCUIntdReMotTqValid','23','1','BE','unsigned','Standard','0','1','0','0','1';'VCU_02_CRC','56','8','BE','unsigned','Standard','0','1','0','0','255';'VCU_02_MsgCntr','48','4','BE','unsigned','Standard','0','1','0','0','15'}  IDPort=off  TimestampPort=off  ErrorPort=off  RemotePort=off  LengthPort=off  StatusPort=off  ApplyMinMax=off
      settings: DataFormat=CANdb specified signals
  Terminator{1..4} (4 alike) : Terminator
  wires:
  In1/1 -> Chassis 1 VCU_02/1
  Chassis 1 VCU_02/1 -> Terminator1/1  "VCU_02_AccrPedlActPosn"
  Chassis 1 VCU_02/3 -> Terminator2/1  "VCU_02_AccrPedlEfcPosn"
  Chassis 1 VCU_02/6 -> Terminator3/1  "VCU_02_IntdFrntMotTq"
  Chassis 1 VCU_02/8 -> Terminator4/1  "VCU_02_IntdReMotTq"

== system mVeh_fun_tbm/cu_tbm/Height Snr/Subsystem/Height Snr ==
  In1 : Inport  OutDataTypeStr=single
  Height Snr : canmsglib/CAN Unpack  CANdbFile=C:\Users\bowen.zheng\Desktop\spdGoat_prj_20230605\spdGoat_prj_20230605\support\dbc\HF-500C Sensor.dbc  MsgList=DataFrame_HF500C  MsgName=DataFrame_HF500C  MsgIDType=Standard (11-bit identifier)  MsgIdentifier=2047  MsgLength=8  SignalInfo={'Height','32','16','LE','unsigned','Standard','0','0.01','0','0','750';'SensorType','24','8','LE','unsigned','Standard','0','1','0','0','255';'SerialNo','0','24','LE','unsigned','Standard','0','1','0','0','16777200';'Unused','48','16','LE','unsigned','Standard','0','1','0','0','65535'}  IDPort=off  TimestampPort=on  ErrorPort=off  RemotePort=off  LengthPort=off  StatusPort=off  ApplyMinMax=off
      settings: DataFormat=CANdb specified signals
  Height : Outport
  wires:
  In1/1 -> Height Snr/1
  Height Snr/1 -> Height/1  "snr_H"

== system mVeh_fun_tbm/cu_tbm/PVRR read/Subsystem/PVRR ==
  In1 : Inport
  Bus Creator : BusCreator  Inputs=2
  Bus Creator1 : BusCreator  Inputs=2
  PVRR front : canmsglib/CAN Unpack  CANdbFile=D:\Desktop\spdGoat_prj_20230526\spdGoat_prj_20230526\support\dbc\PVRR.dbc  MsgList=(none)  MsgName=FAST_MEAS_PRESS_FRONT  MsgIDType=Standard (11-bit identifier)  MsgIdentifier=273  MsgLength=4  SignalInfo={'PVRR_Id','8','8','LE','unsigned','Standard','0','1','0','0','255';'PressCounter','0','8','LE','unsigned','Standard','0','1','0','0','255';'Pressure','16','8','LE','unsigned','Standard','0','1.69','69.7','69.7','500.65'}  IDPort=off  TimestampPort=on  ErrorPort=off  RemotePort=off  LengthPort=off  StatusPort=off  ApplyMinMax=off
      settings: DataFormat=CANdb specified signals
  PVRR rear : canmsglib/CAN Unpack  CANdbFile=D:\Desktop\spdGoat_prj_20230526\spdGoat_prj_20230526\support\dbc\PVRR.dbc  MsgList=(none)  MsgName=FAST_MEAS_PRESS_REAR  MsgIDType=Standard (11-bit identifier)  MsgIdentifier=289  MsgLength=4  SignalInfo={'PVRR_Id','8','8','LE','unsigned','Standard','0','1','0','0','255';'PressCounter','0','8','LE','unsigned','Standard','0','1','0','0','255';'Pressure','16','8','LE','unsigned','Standard','0','1.69','69.7','69.7','500.65'}  IDPort=off  TimestampPort=on  ErrorPort=off  RemotePort=off  LengthPort=off  StatusPort=off  ApplyMinMax=off
      settings: DataFormat=CANdb specified signals
  Terminator : Terminator
  Terminator1 : Terminator
  PVRR_press : Outport
  PVRR_timestamp : Outport  Port=2
  wires:
  PVRR rear/3 -> Bus Creator/2  "PVRR_press_rear"
  In1/1 -> PVRR rear/1, PVRR front/1
  PVRR rear/4 -> Bus Creator1/2  "PVRR_timestamp_rear"
  PVRR front/3 -> Bus Creator/1  "PVRR_press_front"
  PVRR front/4 -> Bus Creator1/1  "PVRR_timestamp_front"
  Bus Creator/1 -> PVRR_press/1
  PVRR front/1 -> Terminator1/1  "PVRR_front_ID"
  PVRR rear/1 -> Terminator/1  "PVRR_rear_ID"
  Bus Creator1/1 -> PVRR_timestamp/1

== system mVeh_fun_tbm/cu_tbm/Sensata  Read/Subsystem/TPMS_TireBurst_Matrix ==
  In1 : Inport
  Bus Creator : BusCreator  Inputs=4
  Bus Creator1 : BusCreator  Inputs=4
  Bus Creator2 : BusCreator  Inputs=2
  TPMS_TireBurst : canmsglib/CAN Unpack  CANdbFile=.\support\dbc\TBM_mix.dbc  MsgList=TMPS_TireBurst_Msg  MsgName=TMPS_TireBurst_Msg  MsgIDType=Standard (11-bit identifier)  MsgIdentifier=337  MsgLength=8  SignalInfo={'LF_burst_flag','15','1','LE','unsigned','Standard','0','1','0','-Inf','Inf';'LF_burst_pressure','0','8','LE','unsigned','Standard','0','2.5','-2.5','-2.5','632.5';'LF_reserved','8','7','LE','unsigned','Standard','0','1','0','-Inf','Inf';'LR_burst_flag','31','1','LE','unsigned','Standard','0','1','0','-Inf','Inf';'LR_burst_pressure','16','8','LE','unsigned','Standard','0','2.5','-2.5','-2.5','632.5';'LR_reserved','24','7','LE','unsigned','Standard','0','1','0','-Inf','Inf';'RF_burst_flag','63','1','LE','unsigned','Standard','0','1','0','-Inf','Inf';'RF_burst_pressure','48','8','LE','unsigned','Standard','0','2.5','-2.5','-2.5','632.5';'RF_reserved','56','7','LE','unsigned','Standard','0','1','0','-Inf','Inf';'RR_burst_flag','47','1','LE','unsigned','Standard','0','1','0','-Inf','Inf';'RR_burst_pressure','32','8','LE','unsigned','Standard','0','2.5','-2.5','-2.5','632.5';'RR_reserved','40','7','LE','unsigned','Standard','0','1','0','-Inf','Inf'}  IDPort=off  TimestampPort=off  ErrorPort=off  RemotePort=off  LengthPort=off  StatusPort=off  ApplyMinMax=off
      settings: DataFormat=CANdb specified signals
  TPMS_TireBurst1 : canmsglib/CAN Unpack  CANdbFile=.\support\dbc\TBM_mix.dbc  MsgList=TPMS_01  MsgName=TPMS_01  MsgIDType=Extended (29-bit identifier)  MsgIdentifier=419423795  MsgLength=8  SignalInfo={'Sensor_ID_Prog_Status','56','2','LE','unsigned','Standard','0','1','0','0','3';'Tyre_Over_Temp_Status','48','2','LE','unsigned','Standard','0','1','0','0','3';'Tyre_Pressure','16','10','LE','unsigned','Standard','0','2','0','0','2046';'Tyre_Pressure_Status','42','4','LE','unsigned','Standard','0','1','0','0','15';'Tyre_Temperature','8','8','LE','unsigned','Standard','0','1','-40','-40','215';'WU_Battery_Status','26','4','LE','unsigned','Standard','0','10','0','0','150';'Wheel_Location_ID','0','8','LE','unsigned','Standard','0','1','0','0','255'}  IDPort=off  TimestampPort=off  ErrorPort=off  RemotePort=off  LengthPort=off  StatusPort=off  ApplyMinMax=off
      settings: DataFormat=CANdb specified signals
  TPMS_TireBurst2 : canmsglib/CAN Unpack  CANdbFile=.\support\dbc\TBM_mix.dbc  MsgList=CM3  MsgName=CM3  MsgIDType=Extended (29-bit identifier)  MsgIdentifier=419288097  MsgLength=8  SignalInfo={'KeySwitchIgnitionPower','20','2','LE','unsigned','Standard','0','1','0','0','3'}  IDPort=off  TimestampPort=off  ErrorPort=off  RemotePort=off  LengthPort=off  StatusPort=off  ApplyMinMax=off
      settings: DataFormat=CANdb specified signals
  Terminator : Terminator
  Terminator1 : Terminator
  TPMS_TireBurst*1 : Outport
  wires:
  In1/1 -> TPMS_TireBurst2/1, TPMS_TireBurst1/1, TPMS_TireBurst/1
  TPMS_TireBurst/1 -> Bus Creator1/1  "LF_burst_flag"
  TPMS_TireBurst/2 -> Bus Creator/1  "LF_burst_pressure"
  TPMS_TireBurst/4 -> Bus Creator1/3  "LR_burst_flag"
  TPMS_TireBurst/5 -> Bus Creator/3  "LR_burst_pressure"
  TPMS_TireBurst/11 -> Bus Creator/4  "RR_burst_pressure"
  TPMS_TireBurst/10 -> Bus Creator1/4  "RR_burst_flag"
  TPMS_TireBurst/8 -> Bus Creator/2  "RF_burst_pressure"
  TPMS_TireBurst/7 -> Bus Creator1/2  "RF_burst_flag"
  Bus Creator1/1 -> Bus Creator2/1  "Sensata_burst_flag"
  Bus Creator/1 -> Bus Creator2/2  "Sensata_burst_pressure"
  Bus Creator2/1 -> TPMS_TireBurst*1/1
  TPMS_TireBurst1/3 -> Terminator/1  "Tyre_Pressure_all"
  TPMS_TireBurst2/1 -> Terminator1/1  "ignition"
